simulink model "simulink_robo_adaptativo_figura1"  (R2014a)
settings: Solver=ode45  StartTime=0.0  StopTime=10.0  RelTol=1e-3
undefined symbols (not defined in the file): a, b, Ic, Kp, L, m, r, trajetoria, Ts, xo
settings Model: Creator=Thiago Lobo  LastModifiedBy=Thiago Lobo

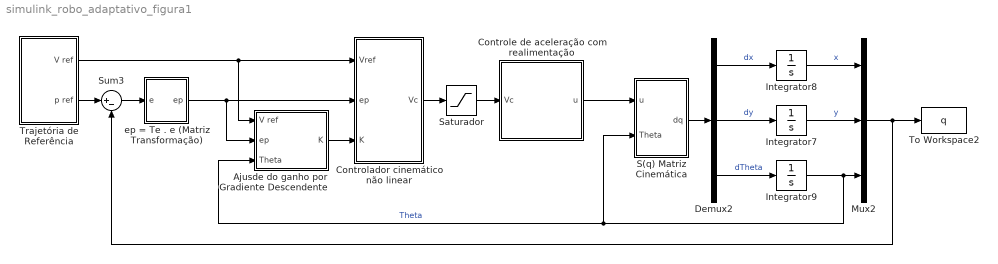
== system simulink_robo_adaptativo_figura1 ==
  "Ajusde do ganho por Gradiente Descendente " : Subsystem
  Controlador cinemático não linear : Subsystem
  Controle de aceleração com realimentação : Subsystem
  Demux2 : Demux  Outputs=3
  Integrator7 : Integrator  InitialCondition=xo
  Integrator8 : Integrator  InitialCondition=xo
  Integrator9 : Integrator  InitialCondition=xo
  Mux2 : Mux  Inputs=3
  S(q) Matriz Cinemática : Subsystem
  Saturador : Saturate  UpperLimit=[0.8 0.8]  LowerLimit=-[0 0.8]
  Sum3 : Sum  Inputs=|+-  SampleTime=Ts
  To Workspace2 : ToWorkspace  VariableName=q  SampleTime=Ts
  Trajetória de Referência : Subsystem
  ep = Te . e (Matriz Transformação) : Subsystem
  wires:
  Sum3/1 -> ep = Te . e (Matriz Transformação)/1(e)
  "Ajusde do ganho por Gradiente Descendente "/1(K) -> Controlador cinemático não linear/3(K)
  ep = Te . e (Matriz Transformação)/1(ep) -> Controlador cinemático não linear/2(ep), "Ajusde do ganho por Gradiente Descendente "/2(ep)
  Trajetória de Referência/2(p ref) -> Sum3/1
  S(q) Matriz Cinemática/1(dq) -> Demux2/1
  Demux2/3 -> Integrator9/1  "dTheta"
  Demux2/2 -> Integrator7/1  "dy"
  Demux2/1 -> Integrator8/1  "dx"
  Integrator8/1 -> Mux2/1  "x"
  Integrator7/1 -> Mux2/2  "y"
  Integrator9/1 -> "Ajusde do ganho por Gradiente Descendente "/3(Theta), S(q) Matriz Cinemática/2(Theta), Mux2/3  "Theta"
  Trajetória de Referência/1(V ref) -> "Ajusde do ganho por Gradiente Descendente "/1(V ref), Controlador cinemático não linear/1(Vref)
  Controlador cinemático não linear/1(Vc) -> Saturador/1
  Mux2/1 -> To Workspace2/1, Sum3/2
  Saturador/1 -> Controle de aceleração com realimentação/1(Vc)
  Controle de aceleração com realimentação/1(u) -> S(q) Matriz Cinemática/1(u)

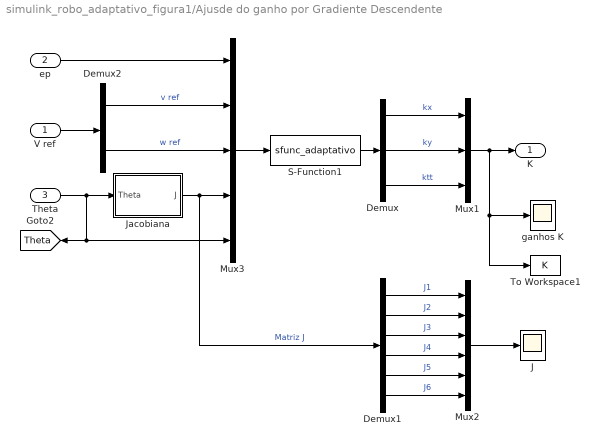
== system simulink_robo_adaptativo_figura1/Ajusde do ganho por Gradiente Descendente  ==
  V ref : Inport
  ep : Inport  Port=2
  Theta : Inport  Port=3
  Demux : Demux  Outputs=3
  Demux1 : Demux  Outputs=6
  Demux2 : Demux  Outputs=2
  J : Scope
      settings: ShowLegends=on  TimeRange=10  SaveName=ScopeData13
  Jacobiana : Subsystem
  Mux1 : Mux  Inputs=3
  Mux2 : Mux  Inputs=6
  Mux3 : Mux  Inputs=5
  S-Function1 : S-Function  FunctionName=sfunc_adaptativo  Parameters=Ts  EnableBusSupport=off
  To Workspace1 : ToWorkspace  VariableName=K  SampleTime=Ts
  ganhos K : Scope
      settings: ShowLegends=on  TimeRange=10  YMin=-100  YMax=220  SaveName=ScopeData14
  K : Outport
  tag scope: Theta=global
  wires:
  Mux3/1 -> S-Function1/1
  S-Function1/1 -> Demux/1
  Demux/3 -> Mux1/3  "ktt"
  Demux/2 -> Mux1/2  "ky"
  Demux/1 -> Mux1/1  "kx"
  ep/1 -> Mux3/1
  Theta/1 -> Mux3/5, [Theta], Jacobiana/1(Theta)
  Jacobiana/1(J) -> Demux1/1, Mux3/4  "Matriz J"
  Demux1/3 -> Mux2/3  "J3"
  Demux1/2 -> Mux2/2  "J2"
  Demux1/1 -> Mux2/1  "J1"
  Demux1/4 -> Mux2/4  "J4"
  Demux1/5 -> Mux2/5  "J5"
  Demux1/6 -> Mux2/6  "J6"
  Mux1/1 -> To Workspace1/1, ganhos K/1, K/1
  Mux2/1 -> J/1
  V ref/1 -> Demux2/1
  Demux2/2 -> Mux3/3  "w ref"
  Demux2/1 -> Mux3/2  "v ref"

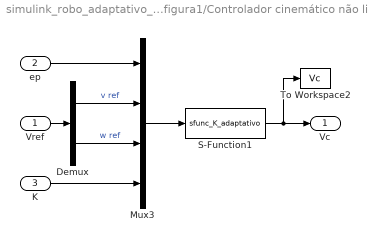
== system simulink_robo_adaptativo_figura1/Controlador cinemático não linear ==
  Vref : Inport
  ep : Inport  Port=2
  K : Inport  Port=3
  Demux : Demux  Outputs=2
  Mux3 : Mux
  S-Function1 : S-Function  FunctionName=sfunc_K_adaptativo  Parameters=Ts  EnableBusSupport=off
  To Workspace2 : ToWorkspace  VariableName=Vc  SampleTime=Ts
  Vc : Outport
  wires:
  Mux3/1 -> S-Function1/1
  Demux/1 -> Mux3/2  "v ref"
  Demux/2 -> Mux3/3  "w ref"
  ep/1 -> Mux3/1
  K/1 -> Mux3/4
  S-Function1/1 -> To Workspace2/1, Vc/1
  Vref/1 -> Demux/1

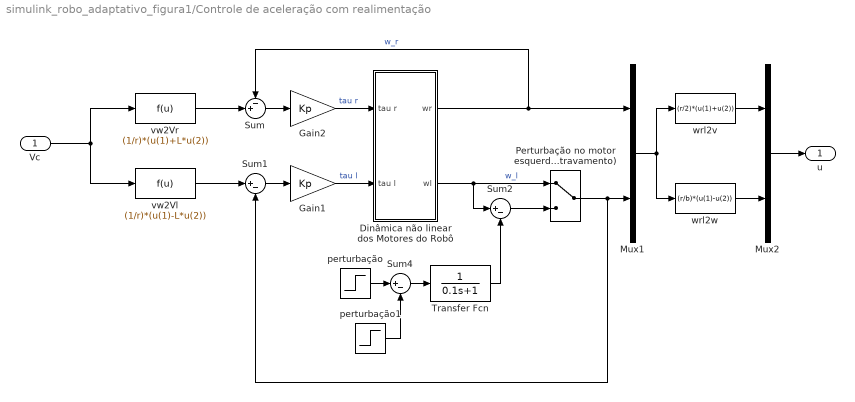
== system simulink_robo_adaptativo_figura1/Controle de aceleração com realimentação ==
  Vc : Inport
  Dinâmica não linear dos Motores do Robô : Subsystem
  Gain1 : Gain  Gain=Kp
  Gain2 : Gain  Gain=Kp
  Mux1 : Mux  Inputs=2
  Mux2 : Mux  Inputs=2
  Perturbação no motor esquerdo (travamento) : ManualSwitch
  Sum : Sum  Inputs=-+|
  Sum1 : Sum  Inputs=|+-
  Sum2 : Sum  Inputs=|+-
  Sum4 : Sum  Inputs=|+-
  Transfer Fcn : TransferFcn  Denominator=[0.1 1]
  perturbação : Step  Time=6  After=5  SampleTime=Ts
  perturbação1 : Step  Time=6.5  After=5  SampleTime=Ts
  vw2Vl : Fcn  Expr=(1/r)*(u(1)-L*u(2))
  vw2Vr : Fcn  Expr=(1/r)*(u(1)+L*u(2))
  wrl2v : Fcn  Expr=(r/2)*(u(1)+u(2))
  wrl2w : Fcn  Expr=(r/b)*(u(1)-u(2))
  u : Outport
  wires:
  Gain2/1 -> Dinâmica não linear dos Motores do Robô/1(tau r)  "tau r"
  Sum/1 -> Gain2/1
  Gain1/1 -> Dinâmica não linear dos Motores do Robô/2(tau l)  "tau l"
  Sum1/1 -> Gain1/1
  Dinâmica não linear dos Motores do Robô/1(wr) -> Sum/1, Mux1/1  "w_r"
  Mux1/1 -> wrl2v/1, wrl2w/1
  wrl2v/1 -> Mux2/1
  wrl2w/1 -> Mux2/2
  vw2Vl/1 -> Sum1/1
  Vc/1 -> vw2Vr/1, vw2Vl/1
  perturbação/1 -> Sum4/1
  perturbação1/1 -> Sum4/2
  Sum4/1 -> Transfer Fcn/1
  Perturbação no motor esquerdo (travamento)/1 -> Sum1/2, Mux1/2
  Transfer Fcn/1 -> Sum2/2
  vw2Vr/1 -> Sum/2
  Dinâmica não linear dos Motores do Robô/2(wl) -> Sum2/1, Perturbação no motor esquerdo (travamento)/1  "w_l"
  Sum2/1 -> Perturbação no motor esquerdo (travamento)/2
  Mux2/1 -> u/1

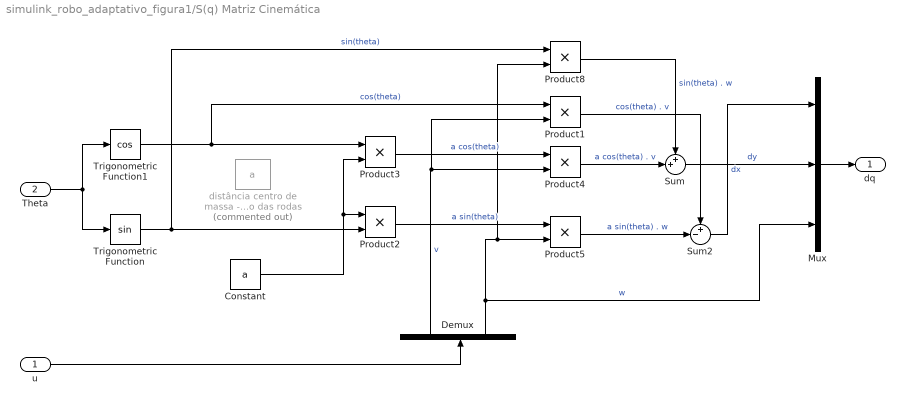
== system simulink_robo_adaptativo_figura1/S(q) Matriz Cinemática ==
  u : Inport
  Theta : Inport  Port=2
  Constant : Constant  Value=a
  Demux : Demux  Outputs=2
  Mux : Mux  Inputs=3
  Product{1..5,8} (6 alike) : Product
  Sum : Sum  Inputs=++|
  Sum2 : Sum  Inputs=+-|
  Trigonometric Function : Trigonometry
  Trigonometric Function1 : Trigonometry  Operator=cos
  distância centro de massa - eixo das rodas : FromWorkspace  Commented=on  VariableName=a  SampleTime=Ts
  dq : Outport
  wires:
  Theta/1 -> Trigonometric Function1/1, Trigonometric Function/1
  Demux/2 -> Mux/3, Product5/2, Product8/2  "w"
  u/1 -> Demux/1
  Mux/1 -> dq/1
  Product2/1 -> Product5/1  "a sin(theta)"
  Product3/1 -> Product4/1  "a cos(theta)"
  Product5/1 -> Sum2/2  "a sin(theta) . w"
  Trigonometric Function/1 -> Product2/2, Product8/1  "sin(theta)"
  Trigonometric Function1/1 -> Product1/1, Product3/1  "cos(theta)"
  Product4/1 -> Sum/2  "a cos(theta) . v"
  Demux/1 -> Product4/2, Product1/2  "v"
  Product1/1 -> Sum2/1  "cos(theta) . v"
  Product8/1 -> Sum/1  "sin(theta) . w"
  Sum/1 -> Mux/2  "dy"
  Sum2/1 -> Mux/1  "dx"
  Constant/1 -> Product3/2, Product2/1

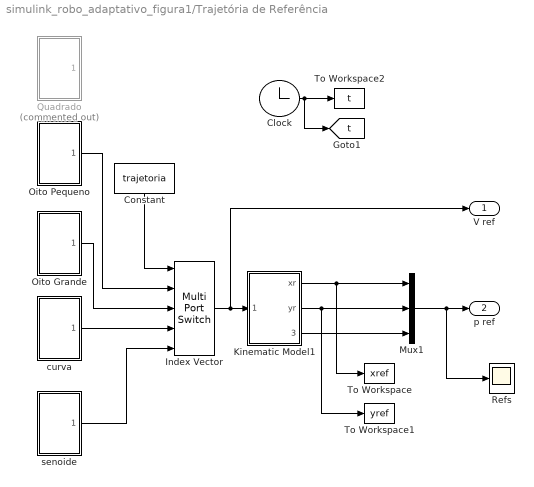
== system simulink_robo_adaptativo_figura1/Trajetória de Referência ==
  Clock : Clock
  Constant : Constant  Value=trajetoria  SampleTime=Ts
  Index Vector : MultiPortSwitch  DataPortOrder=Specify indices  Inputs=1  DataPortIndices={1,2,3,4}
  Kinematic Model1 : Subsystem
  Mux1 : Mux  Inputs=3
  Oito Grande : Subsystem
  Oito Pequeno : Subsystem
  Quadrado : Subsystem  Commented=on
  Refs : Scope
      settings: ShowLegends=on  TimeRange=10  SaveName=ScopeData12
  To Workspace : ToWorkspace  VariableName=xref  SampleTime=Ts
  To Workspace1 : ToWorkspace  VariableName=yref  SampleTime=Ts
  To Workspace2 : ToWorkspace  VariableName=t  SampleTime=Ts
  curva : Subsystem
  senoide : Subsystem
  V ref : Outport
  p ref : Outport  Port=2
  tag scope: t=global
  wires:
  Kinematic Model1/1(xr) -> To Workspace/1, Mux1/1
  Kinematic Model1/3(thetar) -> Mux1/3
  Mux1/1 -> Refs/1, p ref/1
  Kinematic Model1/2(yr) -> To Workspace1/1, Mux1/2
  Index Vector/1 -> V ref/1, Kinematic Model1/1(vw_ref)
  Constant/1 -> Index Vector/1
  senoide/1(vw_ref) -> Index Vector/5
  Oito Grande/1(vw_ref) -> Index Vector/3
  Oito Pequeno/1(vw_ref) -> Index Vector/2
  curva/1(vw_ref) -> Index Vector/4
  Clock/1 -> To Workspace2/1, [t]

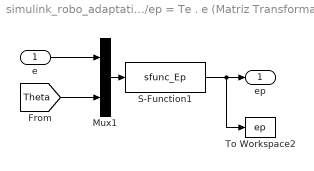
== system simulink_robo_adaptativo_figura1/ep = Te . e (Matriz Transformação) ==
  e : Inport
  Mux1 : Mux  Inputs=2
  S-Function1 : S-Function  FunctionName=sfunc_Ep  Parameters=Ts  EnableBusSupport=off
  To Workspace2 : ToWorkspace  VariableName=ep  SampleTime=Ts
  ep : Outport
  wires:
  S-Function1/1 -> To Workspace2/1, ep/1
  Mux1/1 -> S-Function1/1
  e/1 -> Mux1/1
  [Theta] -> Mux1/2

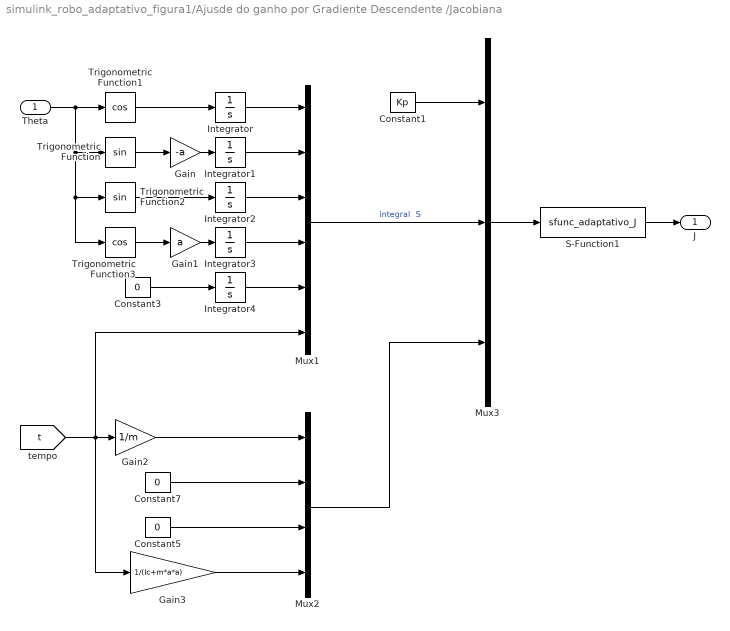
== system simulink_robo_adaptativo_figura1/Ajusde do ganho por Gradiente Descendente /Jacobiana ==
  Theta : Inport
  Constant1 : Constant  Value=Kp  SampleTime=Ts
  Constant3 : Constant  Value=0  SampleTime=Ts
  Constant5 : Constant  Value=0  SampleTime=Ts
  Constant7 : Constant  Value=0  SampleTime=Ts
  Gain : Gain  Gain=-a
  Gain1 : Gain  Gain=a
  Gain2 : Gain  Gain=1/m
  Gain3 : Gain  Gain=1/(Ic+m*a*a)
  Integrator{,1..4} (5 alike) : Integrator
  Mux1 : Mux  Inputs=6
  Mux2 : Mux
  Mux3 : Mux  Inputs=3
  S-Function1 : S-Function  FunctionName=sfunc_adaptativo_J  Parameters=Ts  EnableBusSupport=off
  Trigonometric Function : Trigonometry
  Trigonometric Function1 : Trigonometry  Operator=cos
  Trigonometric Function2 : Trigonometry
  Trigonometric Function3 : Trigonometry  Operator=cos
  J : Outport
  wires:
  Mux3/1 -> S-Function1/1
  S-Function1/1 -> J/1
  Constant3/1 -> Integrator4/1
  Trigonometric Function1/1 -> Integrator/1
  Integrator/1 -> Mux1/1
  Integrator2/1 -> Mux1/3
  Integrator3/1 -> Mux1/4
  Integrator4/1 -> Mux1/5
  Integrator1/1 -> Mux1/2
  Gain2/1 -> Mux2/1
  Constant5/1 -> Mux2/3
  Gain3/1 -> Mux2/4
  Constant7/1 -> Mux2/2
  [t] -> Gain2/1, Mux1/6, Gain3/1
  Trigonometric Function/1 -> Gain/1
  Gain/1 -> Integrator1/1
  Theta/1 -> Trigonometric Function1/1, Trigonometric Function/1, Trigonometric Function2/1, Trigonometric Function3/1
  Trigonometric Function2/1 -> Integrator2/1
  Trigonometric Function3/1 -> Gain1/1
  Gain1/1 -> Integrator3/1
  Constant1/1 -> Mux3/1
  Mux1/1 -> Mux3/2  "integral  S"
  Mux2/1 -> Mux3/3

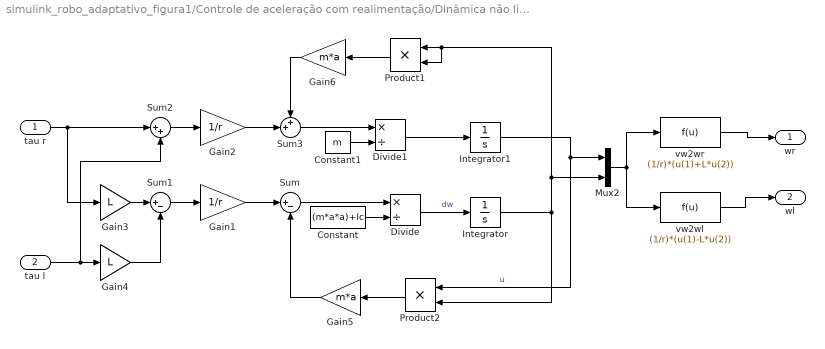
== system simulink_robo_adaptativo_figura1/Controle de aceleração com realimentação/Dinâmica não linear dos Motores do Robô ==
  tau r : Inport
  tau l : Inport  Port=2
  Constant : Constant  Value=(m*a*a)+Ic
  Constant1 : Constant  Value=m
  Divide : Product  Inputs=*/
  Divide1 : Product  Inputs=*/
  Gain1 : Gain  Gain=1/r
  Gain2 : Gain  Gain=1/r
  Gain3 : Gain  Gain=L
  Gain4 : Gain  Gain=L
  Gain5 : Gain  Gain=m*a
  Gain6 : Gain  Gain=m*a
  Integrator : Integrator
  Integrator1 : Integrator
  Mux2 : Mux  Inputs=2
  Product1 : Product  SampleTime=Ts
  Product2 : Product  SampleTime=Ts
  Sum : Sum  Inputs=|+-
  Sum1 : Sum  Inputs=|+-
  Sum2 : Sum  Inputs=|++
  Sum3 : Sum  Inputs=++|
  vw2wl : Fcn  Expr=(1/r)*(u(1)-L*u(2))
  vw2wr : Fcn  Expr=(1/r)*(u(1)+L*u(2))
  wr : Outport
  wl : Outport  Port=2
  wires:
  Divide/1 -> Integrator/1  "dw"
  tau l/1 -> Sum2/2, Gain4/1
  Integrator/1 -> Mux2/2, Product1/1, Product1/2, Product2/2
  tau r/1 -> Gain3/1, Sum2/1
  Gain3/1 -> Sum1/1
  Gain4/1 -> Sum1/2
  Sum1/1 -> Gain1/1
  Integrator1/1 -> Mux2/1, Product2/1  "u"
  Product2/1 -> Gain5/1
  Sum/1 -> Divide/1
  Constant/1 -> Divide/2
  Gain1/1 -> Sum/1
  Gain5/1 -> Sum/2
  Sum2/1 -> Gain2/1
  Gain2/1 -> Sum3/2
  Product1/1 -> Gain6/1
  Gain6/1 -> Sum3/1
  Divide1/1 -> Integrator1/1
  Sum3/1 -> Divide1/1
  Constant1/1 -> Divide1/2
  vw2wr/1 -> wr/1
  vw2wl/1 -> wl/1
  Mux2/1 -> vw2wr/1, vw2wl/1

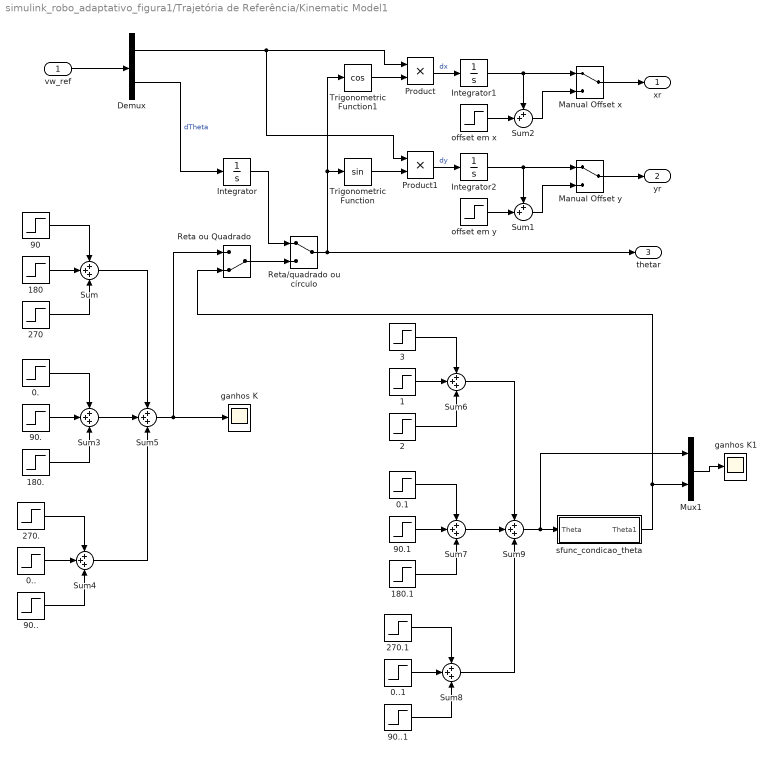
== system simulink_robo_adaptativo_figura1/Trajetória de Referência/Kinematic Model1 ==
  vw_ref : Inport
  0. : Step  Time=80  After=-3*pi/2  SampleTime=Ts
  0.. : Step  Time=160  After=-3*pi/2  SampleTime=Ts
  0..1 : Step  Time=160  After=-3*pi/2  SampleTime=Ts
  0.1 : Step  Time=80  After=-3*pi/2  SampleTime=Ts
  1 : Step  Time=40  After=pi/2  SampleTime=Ts
  180 : Step  Time=40  After=pi/2  SampleTime=Ts
  180. : Step  Time=120  After=pi/2  SampleTime=Ts
  180.1 : Step  Time=120  After=pi/2  SampleTime=Ts
  2 : Step  Time=60  After=pi/2  SampleTime=Ts
  270 : Step  Time=60  After=pi/2  SampleTime=Ts
  270. : Step  Time=140  After=pi/2  SampleTime=Ts
  270.1 : Step  Time=140  After=pi/2  SampleTime=Ts
  3 : Step  Time=20  After=pi/2  SampleTime=Ts
  90 : Step  Time=20  After=pi/2  SampleTime=Ts
  90. : Step  Time=100  After=pi/2  SampleTime=Ts
  90.. : Step  Time=180  After=pi/2  SampleTime=Ts
  90..1 : Step  Time=180  After=pi/2  SampleTime=Ts
  90.1 : Step  Time=100  After=pi/2  SampleTime=Ts
  Demux : Demux  Outputs=2
  Integrator : Integrator
  Integrator1 : Integrator
  Integrator2 : Integrator
  Manual Offset x : ManualSwitch
  Manual Offset y : ManualSwitch
  Mux1 : Mux  Inputs=2
  Product : Product
  Product1 : Product
  Reta ou Quadrado : ManualSwitch  CurrentSetting=0
  Reta/quadrado ou círculo : ManualSwitch
  Sum{,3..9} (8 alike) : Sum  Inputs=+++
  Sum1 : Sum  Inputs=++|
  Sum2 : Sum  Inputs=++|
  Trigonometric Function : Trigonometry
  Trigonometric Function1 : Trigonometry  Operator=cos
  ganhos K : Scope
      settings: ShowLegends=on  TimeRange=10  YMin=-100  YMax=220  SaveName=ScopeData2
  ganhos K1 : Scope
      settings: ShowLegends=on  TimeRange=10  YMin=1.5708  YMax=1.5708  SaveName=ScopeData4
  offset em x : Step  Time=0  Before=0.5  After=0.5  SampleTime=Ts
  offset em y : Step  Time=0  Before=0.5  After=0.5  SampleTime=Ts
  sfunc_condicao_theta : Subsystem
  xr : Outport
  yr : Outport  Port=2
  thetar : Outport  Port=3
  wires:
  Trigonometric Function1/1 -> Product/2
  Product/1 -> Integrator1/1  "dx"
  Integrator/1 -> Reta/quadrado ou círculo/1
  Product1/1 -> Integrator2/1  "dy"
  Trigonometric Function/1 -> Product1/2
  Demux/1 -> Product/1, Product1/1
  Demux/2 -> Integrator/1  "dTheta"
  vw_ref/1 -> Demux/1
  180/1 -> Sum/2
  270/1 -> Sum/3
  Reta/quadrado ou círculo/1 -> Trigonometric Function1/1, Trigonometric Function/1, thetar/1
  90/1 -> Sum/1
  Integrator2/1 -> Sum1/1, Manual Offset y/1
  Reta ou Quadrado/1 -> Reta/quadrado ou círculo/2
  Manual Offset y/1 -> yr/1
  offset em y/1 -> Sum1/2
  Sum1/1 -> Manual Offset y/2
  Integrator1/1 -> Sum2/1, Manual Offset x/1
  offset em x/1 -> Sum2/2
  Sum2/1 -> Manual Offset x/2
  Manual Offset x/1 -> xr/1
  90./1 -> Sum3/2
  180./1 -> Sum3/3
  0./1 -> Sum3/1
  0../1 -> Sum4/2
  90../1 -> Sum4/3
  270./1 -> Sum4/1
  Sum3/1 -> Sum5/2
  Sum4/1 -> Sum5/3
  Sum/1 -> Sum5/1
  Sum5/1 -> Reta ou Quadrado/1, ganhos K/1
  1/1 -> Sum6/2
  2/1 -> Sum6/3
  3/1 -> Sum6/1
  90.1/1 -> Sum7/2
  180.1/1 -> Sum7/3
  0.1/1 -> Sum7/1
  0..1/1 -> Sum8/2
  90..1/1 -> Sum8/3
  270.1/1 -> Sum8/1
  Sum7/1 -> Sum9/2
  Sum8/1 -> Sum9/3
  Sum6/1 -> Sum9/1
  Sum9/1 -> Mux1/1, sfunc_condicao_theta/1(Theta)
  sfunc_condicao_theta/1(Theta1) -> Reta ou Quadrado/2, Mux1/2
  Mux1/1 -> ganhos K1/1

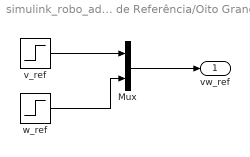
== system simulink_robo_adaptativo_figura1/Trajetória de Referência/Oito Grande ==
  Mux : Mux  Inputs=2
  v_ref : Step  Time=0  Before=0.1  After=0.1  SampleTime=Ts
  w_ref : Step  Time=1200  Before=0.005  After=-0.005  SampleTime=Ts
  vw_ref : Outport
  wires:
  v_ref/1 -> Mux/1
  w_ref/1 -> Mux/2
  Mux/1 -> vw_ref/1

== system simulink_robo_adaptativo_figura1/Trajetória de Referência/Oito Pequeno ==
  Mux : Mux  Inputs=2
  v_ref : Step  Time=0  Before=0.5  After=0.5  SampleTime=Ts
  w_ref : Step  Time=12.5  Before=0.5  After=-0.5  SampleTime=Ts
  vw_ref : Outport
  wires:
  v_ref/1 -> Mux/1
  w_ref/1 -> Mux/2
  Mux/1 -> vw_ref/1

== system simulink_robo_adaptativo_figura1/Trajetória de Referência/Quadrado ==
  Mux : Mux  Inputs=2
  vref : Constant  Value=0.1  SampleTime=Ts
  wref : Constant  Value=0  SampleTime=Ts
  vw_ref : Outport
  wires:
  vref/1 -> Mux/1
  wref/1 -> Mux/2
  Mux/1 -> vw_ref/1

== system simulink_robo_adaptativo_figura1/Trajetória de Referência/curva ==
  Mux : Mux  Inputs=2
  v_ref : Step  Time=0  Before=0.1  After=0.1  SampleTime=Ts
  w_ref : Step  Time=30  Before=0.05  After=-0.05  SampleTime=Ts
  vw_ref : Outport
  wires:
  v_ref/1 -> Mux/1
  w_ref/1 -> Mux/2
  Mux/1 -> vw_ref/1

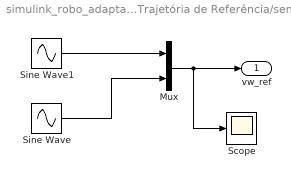
== system simulink_robo_adaptativo_figura1/Trajetória de Referência/senoide ==
  Mux : Mux  Inputs=2
  Scope : Scope
  Sine Wave : Sin  Amplitude=0.1  SampleTime=0
  Sine Wave1 : Sin  Amplitude=0.9  Bias=0.1  Frequency=0.09  SampleTime=0
  vw_ref : Outport
  wires:
  Sine Wave1/1 -> Mux/1
  Sine Wave/1 -> Mux/2
  Mux/1 -> Scope/1, vw_ref/1

== system simulink_robo_adaptativo_figura1/Trajetória de Referência/Kinematic Model1/sfunc_condicao_theta ==
  Theta : Inport
  S-Function1 : S-Function  FunctionName=sfunc_condicao_theta_ref  Parameters=Ts  EnableBusSupport=off
  Theta1 : Outport
  wires:
  S-Function1/1 -> Theta1/1
  Theta/1 -> S-Function1/1
